simulink model "nnpid"  (R2024a)
settings: Solver=VariableStepAuto  StartTime=0.0  StopTime=20  RelTol=1e-3
settings Model: Creator=ericliu  LastModifiedBy=Eason

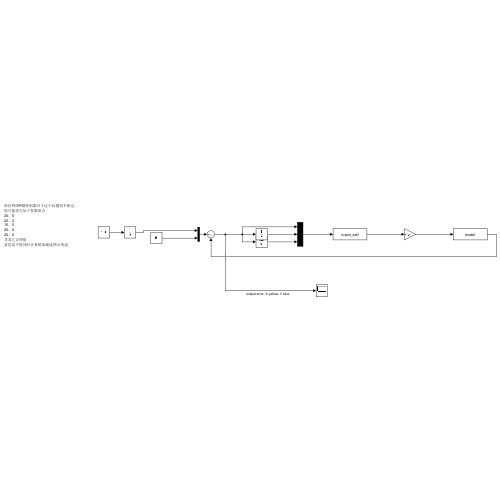
[thumbnail: Simulink's stored preview of the top-level diagram]
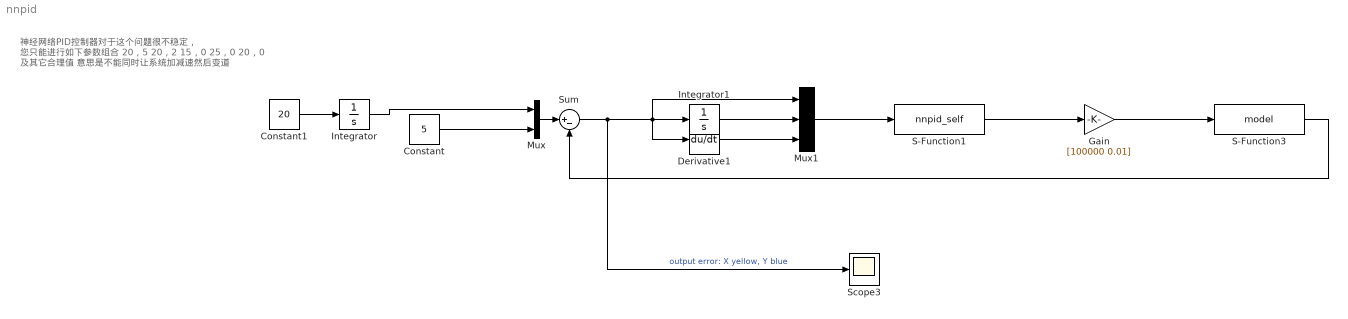
== system nnpid ==
  note: 神经网络PID控制器对于这个问题很不稳定，
      | 您只能进行如下参数组合
      | 20，5
      | 20，2
      | 15，0
      | 25，0
      | 20，0
      | 及其它合理值
      | 意思是不能同时让系统加减速然后变道
  Constant : Constant  Value=5  SampleTime=-1
  Constant1 : Constant  Value=20  SampleTime=-1
  Derivative1 : Derivative
  Gain : Gain  Gain=[100000 0.01]
  Integrator : Integrator
  Integrator1 : Integrator
  Mux : Mux  Inputs=2
  Mux1 : Mux  Inputs=3
  S-Function1 : S-Function  FunctionName=nnpid_self  SFunctionDeploymentMode=off  EnableBusSupport=off
  S-Function3 : S-Function  FunctionName=model  SFunctionDeploymentMode=off  EnableBusSupport=off
  Scope3 : Scope
  Sum : Sum  Inputs=|+-
  wires:
  Constant1/1 -> Integrator/1
  Constant/1 -> Mux/2
  S-Function3/1 -> Sum/2
  S-Function1/1 -> Gain/1
  Mux/1 -> Sum/1
  Sum/1 -> Scope3/1, Derivative1/1, Integrator1/1, Mux1/1  "output error: X yellow, Y blue"
  Mux1/1 -> S-Function1/1
  Derivative1/1 -> Mux1/3
  Gain/1 -> S-Function3/1
  Integrator1/1 -> Mux1/2
  Integrator/1 -> Mux/1
